simulink model "lab7_metoda_releului_slx"  (R2023b)
settings: Solver=ode45  StartTime=0.0  StopTime=50  RelTol=1e-5
settings Model: Creator=Daniela  LastModifiedBy=Daniela

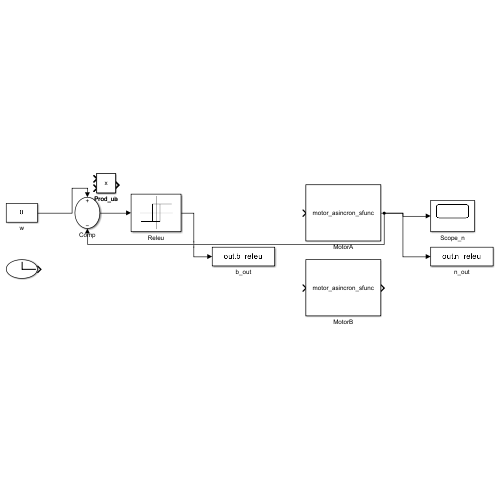
[thumbnail: Simulink's stored preview of the top-level diagram]
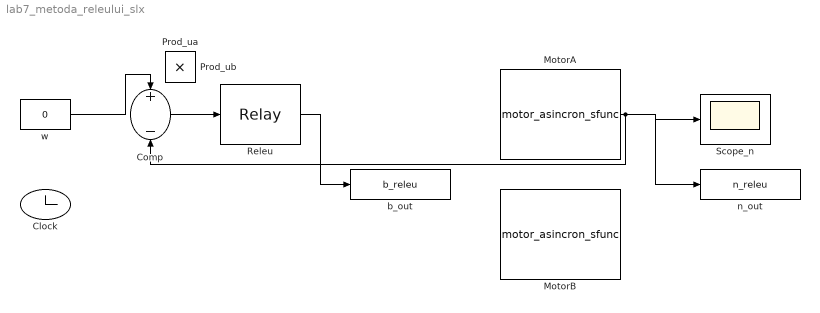
== system lab7_metoda_releului_slx ==
  Clock : Clock
  Comp : Sum  Inputs=+-
  MotorA : M-S-Function  FunctionName=motor_asincron_sfunc
  MotorB : M-S-Function  FunctionName=motor_asincron_sfunc
  Prod_ua : Product
  Prod_ub : Product
  Releu : Relay  OnSwitchValue=50  OffSwitchValue=-50  OffOutputValue=-1
  Scope_n : Scope
  b_out : ToWorkspace  VariableName=b_releu  SampleTime=-1
  n_out : ToWorkspace  VariableName=n_releu  SampleTime=-1
  w : Constant  Value=0
  wires:
  w/1 -> Comp/1
  Comp/1 -> Releu/1
  Releu/1 -> b_out/1
  MotorA/1 -> Scope_n/1, n_out/1, Comp/2
